simulink model "complex_UIO_3"  (R2019b)
settings: Solver=FixedStepAuto  StartTime=0.0  StopTime=60  FixedStep=0.1  RelTol=1e-3
values from neighbouring files (symbols this model uses):
  Ac = [real(A) -imag(A);imag(A) real(A)]    [DAC_UIO_Comp.m]    (also in LinearND_QUANTUM_2020_11_14_2.m = [realA -imagA;imagA realA]; UIO_alternative_2021_01_26.m; UIO_alternative_PAPER_2021_02_17.m = Abar(2:3,2:3); UIO_alternative_PAPER_2021_03_01.m = Abar(2:3,2:3))
  Amc = [real(Am) -imag(Am);imag(Am) real(Am)]    [DAC_UIO_Comp.m]    (also in UIO_alternative_2021_01_26.m)
  Bc = [real(B) -imag(B);imag(B) real(B)]    [DAC_UIO_Comp.m]    (also in UIO_alternative_2021_01_26.m; UIO_alternative_PAPER_2021_02_17.m = Bbar(2:3,:); UIO_alternative_PAPER_2021_03_01.m = Bbar(2:3,:))
  C = double(subs(C_sym,{ep},{0.1}))    [DAC_UIO_Comp.m]    (also in UIO_adaptive_example.m = [1 0 0 0 0;0 0 0 1 0; 0 0 0 0 1]; UIO_adaptive_example_2.m = [1 0 0 0;0 1 0 0]; UIO_adaptive_example_EEG_Balas_2ch.m = [1, epsilon]; UIO_adaptive_example_alternative_EEG_ch6.m = ss_c.C)
  g1 = 4+2j    [DAC_UIO_Comp.m]    (also in UIO_adaptive_example_EEG_Balas_2ch.m = 4; UIO_alternative_2021_01_26.m = 2+1j; UIO_alternative_PAPER_2021_02_17.m = 2; UIO_alternative_PAPER_2021_03_01.m = 2)
  g2 = 0    [DAC_UIO_Comp.m]    (also in UIO_adaptive_example_EEG_Balas_2ch.m = -0.3; UIO_alternative_2021_01_26.m; UIO_alternative_PAPER_2021_02_17.m = 1; UIO_alternative_PAPER_2021_03_01.m)
  g3 = 0    [DAC_UIO_Comp.m]    (also in UIO_adaptive_example_EEG_Balas_2ch.m = 0.1; UIO_alternative_2021_01_26.m; UIO_alternative_PAPER_2021_02_17.m = -3; UIO_alternative_PAPER_2021_03_01.m)
  gamma_e = 1    [DAC_UIO_Comp.m]    (also in UIO_adaptive_example_EEG_Balas_2ch.m; UIO_adaptive_example_alternative_EEG_ch6.m = .0001*ones(length(Am),1); UIO_alternative_2021_01_26.m = 0.001; UIO_alternative_PAPER_2021_02_17.m = 0.0001)
  K_u = ones(size(Fu,1),1)    [UIO_adaptive_example_alternative_EEG_ch6.m]    (also in UIO_alternative_2021_01_26.m = [0.215;ku]; UIO_alternative_PAPER_2021_02_17.m = [2;10;-1.6;10]; UIO_alternative_PAPER_2021_03_01.m = -[K_cvx(3:end,:)]; UIO_alternative_PAPER_2021_03_02.m)
settings Model: Creator=Tris  LastModifiedBy=Tris

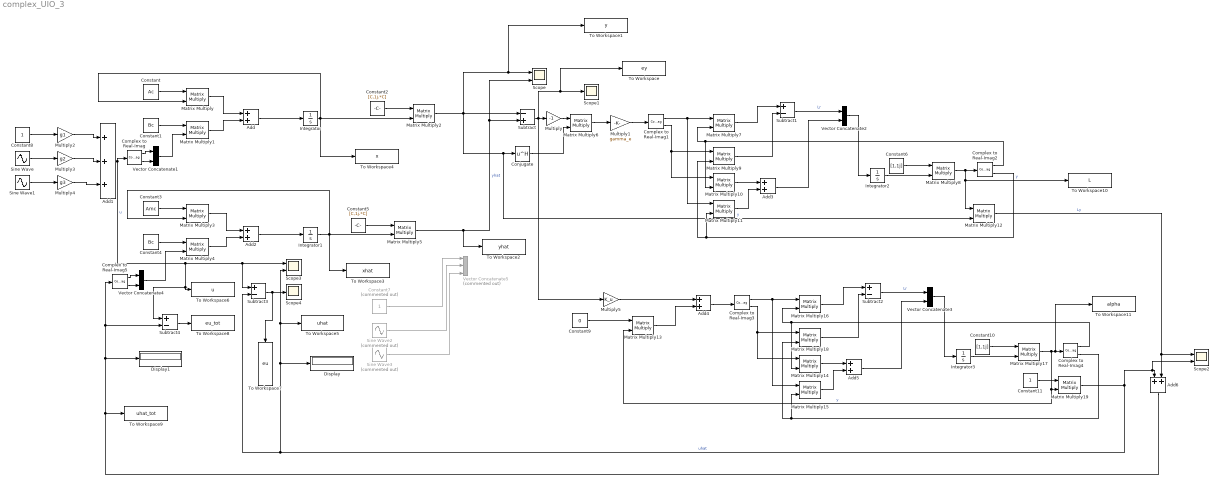
== system complex_UIO_3 ==
  Add{,2..6} (6 alike) : Sum
  Add1 : Sum  Inputs=+++
  Complex to Real-Imag{,1..5} (6 alike) : ComplexToRealImag
  Conjugate : Math  Operator=hermitian  RndMeth=Zero  SaturateOnIntegerOverflow=on
  Constant : Constant  Value=Ac
  Constant1 : Constant  Value=Bc  VectorParams1D=off
  Constant10 : Constant  Value=[1,1j]  VectorParams1D=off
  Constant11 : Constant
  Constant2 : Constant  Value=[C,1j.*C]  VectorParams1D=off
  Constant3 : Constant  Value=Amc
  Constant4 : Constant  Value=Bc  VectorParams1D=off
  Constant5 : Constant  Value=[C,1j.*C]  VectorParams1D=off
  Constant6 : Constant  Value=[1,1j]  VectorParams1D=off
  Constant7 : Constant  Commented=on  VectorParams1D=off
  Constant8 : Constant  VectorParams1D=off
  Constant9 : Constant  Value=0  VectorParams1D=off
  Display : Display
  Display1 : Display
  Integrator : Integrator
  Integrator1 : Integrator
  Integrator2 : Integrator  InitialCondition=[1;0.5]
  Integrator3 : Integrator  InitialCondition=[1;0.5]
  Matrix Multiply{,1..19} (20 alike) : Product  Multiplication=Matrix(*)
  Multiply : Gain  Gain=-1
  Multiply1 : Gain  Gain=gamma_e
  Multiply2 : Gain  Gain=g1
  Multiply3 : Gain  Gain=g2
  Multiply4 : Gain  Gain=g3
  Multiply5 : Gain  Gain=K_u
  Scope : Scope  NumInputPorts=2
  Scope1 : Scope
  Scope2 : Scope  NumInputPorts=2
  Scope3 : Scope  NumInputPorts=2
  Scope4 : Scope
  Sine Wave : Sin  SampleTime=0  VectorParams1D=off
  Sine Wave1 : Sin  Phase=pi/2  SampleTime=0  VectorParams1D=off
  Sine Wave2 : Sin  Commented=on  SampleTime=0  VectorParams1D=off
  Sine Wave3 : Sin  Commented=on  Phase=pi/2  SampleTime=0  VectorParams1D=off
  Subtract : Sum  Inputs=-+
  Subtract{1..4} (4 alike) : Sum  Inputs=+-
  To Workspace : ToWorkspace  VariableName=ey  SaveFormat=Timeseries  SampleTime=-1
  To Workspace1 : ToWorkspace  VariableName=y  SaveFormat=Timeseries  SampleTime=-1
  To Workspace10 : ToWorkspace  VariableName=L  SaveFormat=Timeseries  SampleTime=-1
  To Workspace11 : ToWorkspace  VariableName=alpha  SaveFormat=Timeseries  SampleTime=-1
  To Workspace2 : ToWorkspace  VariableName=yhat  SaveFormat=Timeseries  SampleTime=-1
  To Workspace3 : ToWorkspace  VariableName=xhat  SaveFormat=Timeseries  SampleTime=-1
  To Workspace4 : ToWorkspace  VariableName=x  SaveFormat=Timeseries  SampleTime=-1
  To Workspace5 : ToWorkspace  VariableName=uhat  SaveFormat=Timeseries  SampleTime=-1
  To Workspace6 : ToWorkspace  VariableName=u  SaveFormat=Timeseries  SampleTime=-1
  To Workspace7 : ToWorkspace  VariableName=eu  SaveFormat=Timeseries  SampleTime=-1
  To Workspace8 : ToWorkspace  VariableName=eu_tot  SaveFormat=Timeseries  SampleTime=-1
  To Workspace9 : ToWorkspace  VariableName=uhat_tot  SaveFormat=Timeseries  SampleTime=-1
  Vector Concatenate{1..4} (4 alike) : Concatenate  Mode=Multidimensional array
  Vector Concatenate5 : Concatenate  Commented=on  NumInputs=3  Mode=Multidimensional array
  wires:
  Constant/1 -> Matrix Multiply/1
  Integrator/1 -> Matrix Multiply/2, To Workspace4/1, Matrix Multiply2/2
  Add/1 -> Integrator/1
  Matrix Multiply/1 -> Add/1
  Matrix Multiply1/1 -> Add/2
  Constant1/1 -> Matrix Multiply1/1
  Multiply4/1 -> Add1/3
  Multiply3/1 -> Add1/2
  Multiply2/1 -> Add1/1
  Sine Wave1/1 -> Multiply4/1
  Constant8/1 -> Multiply2/1
  Sine Wave/1 -> Multiply3/1
  Constant2/1 -> Matrix Multiply2/1
  Add1/1 -> Complex to Real-Imag/1, Subtract4/1, To Workspace6/1, Subtract3/1, Scope3/1  "u"
  Complex to Real-Imag/1 -> Vector Concatenate1/1
  Complex to Real-Imag/2 -> Vector Concatenate1/2
  Vector Concatenate1/1 -> Matrix Multiply1/2
  Matrix Multiply2/1 -> To Workspace1/1, Scope/1, Matrix Multiply12/2, Conjugate/1, Subtract/1  "y"
  Constant3/1 -> Matrix Multiply3/1
  Matrix Multiply3/1 -> Add2/1
  Matrix Multiply4/1 -> Add2/2
  Constant4/1 -> Matrix Multiply4/1
  Add2/1 -> Integrator1/1
  Integrator1/1 -> To Workspace3/1, Matrix Multiply5/2, Matrix Multiply3/2
  Constant5/1 -> Matrix Multiply5/1
  Matrix Multiply5/1 -> To Workspace2/1, Subtract/2, Scope/2  "yhat"
  Sine Wave2/1 -> Vector Concatenate5/2
  Sine Wave3/1 -> Vector Concatenate5/3
  Constant7/1 -> Vector Concatenate5/1
  Complex to Real-Imag5/2 -> Vector Concatenate4/2
  Vector Concatenate4/1 -> Matrix Multiply4/2
  Complex to Real-Imag5/1 -> Vector Concatenate4/1
  Subtract/1 -> Multiply5/1, To Workspace/1, Scope1/1, Multiply/1
  Multiply/1 -> Matrix Multiply6/1
  Conjugate/1 -> Matrix Multiply6/2
  Matrix Multiply6/1 -> Multiply1/1
  Add3/1 -> Vector Concatenate2/2
  Matrix Multiply10/1 -> Add3/1
  Subtract1/1 -> Vector Concatenate2/1  "Lr"
  Complex to Real-Imag2/2 -> Matrix Multiply11/2, Matrix Multiply9/2
  Complex to Real-Imag2/1 -> Matrix Multiply7/2, Matrix Multiply10/2
  Matrix Multiply9/1 -> Subtract1/2
  Matrix Multiply11/1 -> Add3/2
  Multiply1/1 -> Complex to Real-Imag1/1
  Complex to Real-Imag1/1 -> Matrix Multiply11/1, Matrix Multiply7/1
  Integrator2/1 -> Matrix Multiply8/2
  Complex to Real-Imag1/2 -> Matrix Multiply10/1, Matrix Multiply9/1
  Matrix Multiply8/1 -> To Workspace10/1, Matrix Multiply12/1, Complex to Real-Imag2/1  "y"
  Matrix Multiply7/1 -> Subtract1/1
  Vector Concatenate2/1 -> Integrator2/1
  Constant6/1 -> Matrix Multiply8/1
  Multiply5/1 -> Add4/1
  Constant9/1 -> Matrix Multiply13/1
  Matrix Multiply13/1 -> Add4/2
  Vector Concatenate3/1 -> Integrator3/1
  Integrator3/1 -> Matrix Multiply17/2
  Complex to Real-Imag3/1 -> Matrix Multiply15/1, Matrix Multiply16/1
  Constant10/1 -> Matrix Multiply17/1
  Matrix Multiply18/1 -> Subtract2/2
  Complex to Real-Imag3/2 -> Matrix Multiply14/1, Matrix Multiply18/1
  Complex to Real-Imag4/2 -> Matrix Multiply15/2, Matrix Multiply18/2
  Subtract2/1 -> Vector Concatenate3/1  "Lr"
  Matrix Multiply14/1 -> Add5/1
  Complex to Real-Imag4/1 -> Matrix Multiply16/2, Matrix Multiply14/2
  Add5/1 -> Vector Concatenate3/2
  Matrix Multiply15/1 -> Add5/2
  Add4/1 -> Complex to Real-Imag3/1
  Matrix Multiply16/1 -> Subtract2/1
  Matrix Multiply17/1 -> Matrix Multiply13/2, Matrix Multiply19/2, To Workspace11/1, Complex to Real-Imag4/1  "y"
  Constant11/1 -> Matrix Multiply19/1
  Matrix Multiply19/1 -> Scope2/2, Add6/1, To Workspace5/1, Scope3/2, Display/1, Subtract3/2  "uhat"
  Matrix Multiply12/1 -> Scope2/1, Add6/2  "Ly"
  Add6/1 -> To Workspace9/1, Subtract4/2, Complex to Real-Imag5/1, Display1/1
  Subtract3/1 -> To Workspace7/1, Scope4/1
  Subtract4/1 -> To Workspace8/1
